simulink model "threephaseinverter"  (R2016a)
settings: Solver=ode4  StartTime=0.0  StopTime=0.1  FixedStep=1e-6  RelTol=1e-3
undefined symbols (not defined in the file): f_sw
libraries: dspsigops x3
settings Model: Creator=Heath  LastModifiedBy=rtw141
settings DataIOCC: LimitDataPoints=on  SaveFormat=Array  SignalLoggingSaveFormat=ModelDataLogs  SignalLoggingName=sigsOut
settings OptimizationCC: ExpressionDepthLimit=2147483647
settings DebuggingCC: SaveWithParameterizedLinksMsg=none  UnderspecifiedInitializationDetection=Classic  MergeDetectMultiDrivingBlocksExec=none  SignalResolutionControl=TryResolveAllWithWarning  MultiTaskDSMMsg=warning  MultiTaskCondExecSysMsg=none  StateNameClashWarn=warning  StrictBusMsg=None
settings HardwareCC: ProdBitPerPointer=32  ProdLargestAtomicFloat=None  ProdIntDivRoundTo=Undefined  ProdEndianess=Unspecified  ProdWordSize=32  ProdHWDeviceType=32-bit Generic  TargetUnknown=on
settings ModelReferenceCC: PropagateSignalLabelsOutOfModel=off
settings GRTTargetCC: CombineOutputUpdateFcns=off  GRTInterface=on
settings ConfigComp: CovModelRefEnable=Off

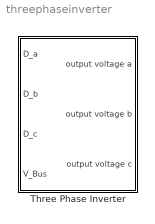
== system threephaseinverter ==
  Three Phase Inverter : Subsystem

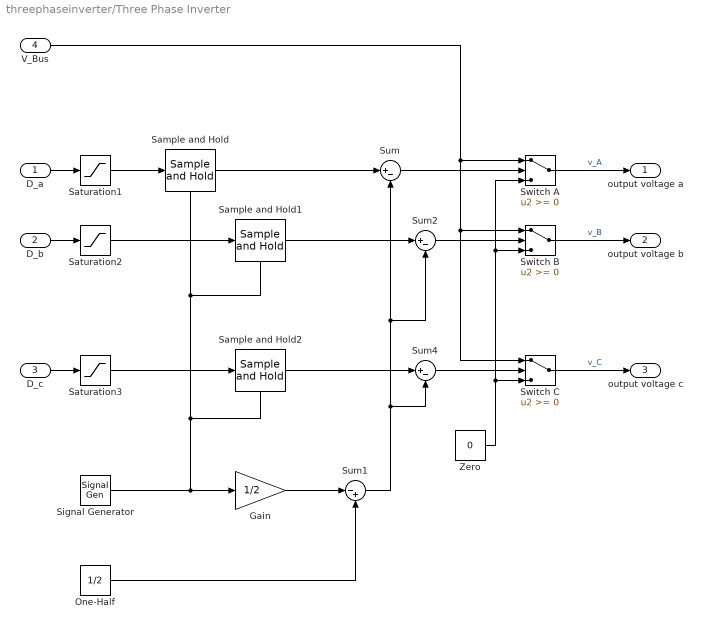
== system threephaseinverter/Three Phase Inverter ==
  D_a : Inport
  D_b : Inport  Port=2
  D_c : Inport  Port=3
  V_Bus : Inport  Port=4
  Gain : Gain  Gain=1/2  SaturateOnIntegerOverflow=on  OutDataTypeStr=Inherit: Same as input  ParamDataTypeStr=Inherit: Same as input
  One-Half : Constant  Value=1/2
  Sample and Hold : dspsigops/Sample and Hold  trig=Falling edge  initCond=0  latchinput=off
  Sample and Hold1 : dspsigops/Sample and Hold  trig=Falling edge  initCond=0  latchinput=off
  Sample and Hold2 : dspsigops/Sample and Hold  trig=Falling edge  initCond=0  latchinput=off
  Saturation1 : Saturate  UpperLimit=1  LowerLimit=0
  Saturation2 : Saturate  UpperLimit=1  LowerLimit=0
  Saturation3 : Saturate  UpperLimit=1  LowerLimit=0
  Signal Generator : SignalGenerator  WaveForm=sawtooth  Frequency=f_sw
  Sum : Sum  Inputs=|+-  SaturateOnIntegerOverflow=on
  Sum1 : Sum  Inputs=|-+  SaturateOnIntegerOverflow=on
  Sum2 : Sum  Inputs=|+-  SaturateOnIntegerOverflow=on
  Sum4 : Sum  Inputs=|+-  SaturateOnIntegerOverflow=on
  Switch A : Switch  SaturateOnIntegerOverflow=on
  Switch B : Switch  SaturateOnIntegerOverflow=on
  Switch C : Switch  SaturateOnIntegerOverflow=on
  Zero : Constant  Value=0
  output voltage a : Outport
  output voltage b : Outport  Port=2
  output voltage c : Outport  Port=3
  wires:
  Sum/1 -> Switch A/2
  Zero/1 -> Switch B/3, Switch A/3, Switch C/3
  Signal Generator/1 -> Sample and Hold/Trigger, Sample and Hold1/Trigger, Sample and Hold2/Trigger, Gain/1
  Gain/1 -> Sum1/1
  One-Half/1 -> Sum1/2
  Sum2/1 -> Switch B/2
  Sum1/1 -> Sum4/2, Sum2/2, Sum/2
  V_Bus/1 -> Switch A/1, Switch B/1, Switch C/1
  D_a/1 -> Saturation1/1
  Sample and Hold/1 -> Sum/1
  D_b/1 -> Saturation2/1
  Sample and Hold1/1 -> Sum2/1
  Saturation1/1 -> Sample and Hold/1
  Saturation2/1 -> Sample and Hold1/1
  D_c/1 -> Saturation3/1
  Saturation3/1 -> Sample and Hold2/1
  Sample and Hold2/1 -> Sum4/1
  Sum4/1 -> Switch C/2
  Switch A/1 -> output voltage a/1  "v_A"
  Switch C/1 -> output voltage c/1  "v_C"
  Switch B/1 -> output voltage b/1  "v_B"
